simulink model "sim_part8"  (R2022b)
settings: Solver=VariableStepAuto  StartTime=0.0  StopTime=15  RelTol=1e-3
undefined symbols (not defined in the file): K61, matA1, matB1
libraries: cstblocks x8
settings Model: Creator=alon  LastModifiedBy=binya
settings SolverCC: AlgebraicLoopSolver=TrustRegion
settings DebuggingCC: UnconnectedInputMsg=warning  UnconnectedOutputMsg=warning  UnconnectedLineMsg=warning  SFMachineParentedDataDiag=warning
settings ModelReferenceCC: EnableRefExpFcnMdlSchedulingChecks=on

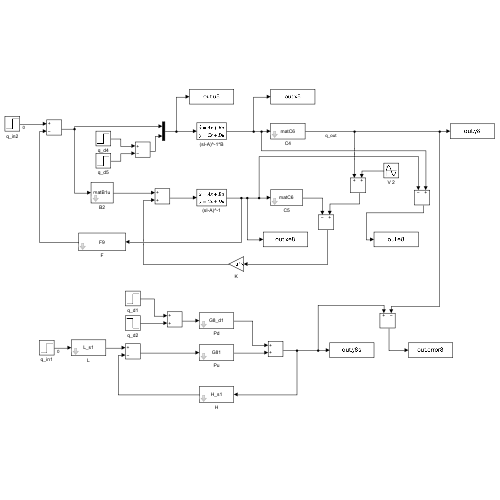
[thumbnail: Simulink's stored preview of the top-level diagram]
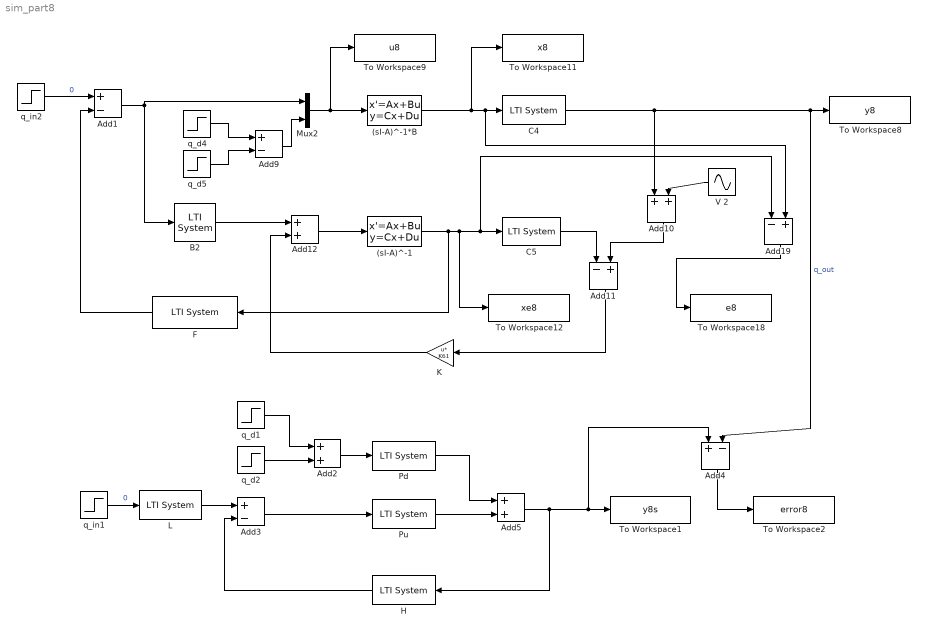
== system sim_part8 ==
  (sI-A)^-1 : StateSpace  A=matA1  B=eye(3)  C=eye(3)  D=[[0 0 0];[0 0 0];[0 0 0]]  InitialCondition=0
  (sI-A)^-1*B : StateSpace  A=matA1  B=matB1  C=eye(3)  D=[[0 0];[0 0];[0 0]]  InitialCondition=0
  Add{1,3..4,9} (4 alike) : Sum  Inputs=+-
  Add{2,5,10,12} (4 alike) : Sum
  Add11 : Sum  Inputs=-+
  Add19 : Sum  Inputs=-+
  B2 : cstblocks/LTI System  sys=matB1u  IC=[]
  C4 : cstblocks/LTI System  sys=matC6  IC=[]
  C5 : cstblocks/LTI System  sys=matC6  IC=[]
  F : cstblocks/LTI System  sys=F9  IC=[]
  H : cstblocks/LTI System  sys=H_s1  IC=[]
  K : Gain  Gain=K61  Multiplication=Matrix(u*K)
  L : cstblocks/LTI System  sys=L_s1  IC=[]
  Mux2 : Mux  Inputs=2
  Pd : cstblocks/LTI System  sys=G8_d1  IC=[]
  Pu : cstblocks/LTI System  sys=G81  IC=[]
  To Workspace1 : ToWorkspace  VariableName=y8s  SaveFormat=Timeseries  SampleTime=-1
  To Workspace11 : ToWorkspace  VariableName=x8  SaveFormat=Timeseries  SampleTime=-1
  To Workspace12 : ToWorkspace  VariableName=xe8  SaveFormat=Timeseries  SampleTime=-1
  To Workspace18 : ToWorkspace  VariableName=e8  SaveFormat=Timeseries  SampleTime=-1
  To Workspace2 : ToWorkspace  VariableName=error8  SaveFormat=Timeseries  SampleTime=-1
  To Workspace8 : ToWorkspace  VariableName=y8  SaveFormat=Timeseries  SampleTime=-1
  To Workspace9 : ToWorkspace  VariableName=u8  SaveFormat=Timeseries  SampleTime=-1
  V 2 : Sin  Amplitude=0  Frequency=10  SampleTime=0
  q_d1 : Step  Time=0  After=12  SampleTime=0
  q_d2 : Step  Time=2.3  After=-12  SampleTime=0
  q_d4 : Step  Time=0  After=12  SampleTime=0
  q_d5 : Step  Time=2.3  After=12  SampleTime=0
  q_in1 : Step  Time=0  After=0  SampleTime=0
  q_in2 : Step  Time=0  After=0  SampleTime=0
  wires:
  Add11/1 -> K/1
  Mux2/1 -> To Workspace9/1, (sI-A)^-1*B/1
  K/1 -> Add12/2
  q_d5/1 -> Add9/2
  V 2/1 -> Add10/2
  q_d4/1 -> Add9/1
  B2/1 -> Add12/1
  (sI-A)^-1*B/1 -> To Workspace11/1, Add19/2, C4/1
  Add12/1 -> (sI-A)^-1/1
  C4/1 -> Add10/1, To Workspace8/1, Add4/2  "q_out"
  Add9/1 -> Mux2/2
  Add19/1 -> To Workspace18/1
  Add10/1 -> Add11/2
  C5/1 -> Add11/1
  (sI-A)^-1/1 -> F/1, Add19/1, C5/1, To Workspace12/1
  F/1 -> Add1/2
  q_in2/1 -> Add1/1  "0"
  Add1/1 -> Mux2/1, B2/1
  q_d2/1 -> Add2/2
  q_d1/1 -> Add2/1
  q_in1/1 -> L/1  "0"
  L/1 -> Add3/1
  H/1 -> Add3/2
  Add4/1 -> To Workspace2/1
  Add5/1 -> H/1, Add4/1, To Workspace1/1
  Pu/1 -> Add5/2
  Pd/1 -> Add5/1
  Add2/1 -> Pd/1
  Add3/1 -> Pu/1
